simulink model "DBL_Master"  (R2020b)
settings: configuration reference "VLS_Standard_Configuration" (kept outside this file)
undefined symbols (not defined in the file): C_CSpeed0, C_DblDeadZone, C_DblInterDblAngValues, C_DblInterStwAngValues, C_DblRateLimit, C_DblSpeed0, C_LeftDblMaxAngle, C_LeftDblMinAngle, C_RightDblMaxAngle, C_RightDblMinAngle
libraries: DBL_MasterLib x1
settings Model: DataDictionary=DBL_Master_DD.sldd  EnableAccessToBaseWorkspace=off  Creator=mteama  LastModifiedBy=ahashem
settings ConfigSetRef: SourceName=VLS_Standard_Configuration

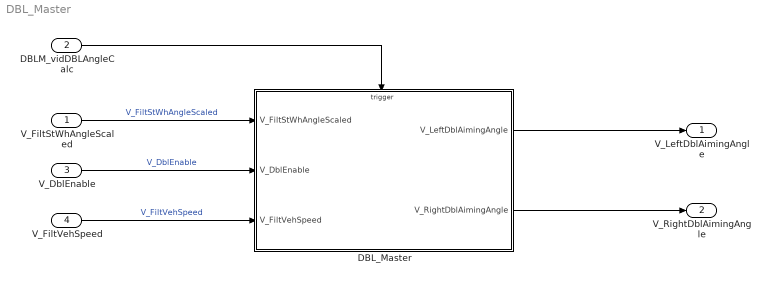
== system DBL_Master ==
  V_FiltStWhAngleScaled : Inport
  DBLM_vidDBLAngleCalc : Inport  Port=2  SampleTime=0.02  OutputFunctionCall=on
  V_DblEnable : Inport  Port=3
  V_FiltVehSpeed : Inport  Port=4
  DBL_Master : Subsystem  Description=DBLMasterLaw2 subsystem  TreatAsAtomicUnit=on
  V_LeftDblAimingAngle : Outport  VectorParamsAs1DForOutWhenUnconnected=off
  V_RightDblAimingAngle : Outport  Port=2  VectorParamsAs1DForOutWhenUnconnected=off
  wires:
  V_FiltStWhAngleScaled/1 -> DBL_Master/1(V_FiltStWhAngleScaled)  "V_FiltStWhAngleScaled"
  DBL_Master/1(V_LeftDblAimingAngle) -> V_LeftDblAimingAngle/1
  DBLM_vidDBLAngleCalc/1 -> DBL_Master/Trigger
  V_DblEnable/1 -> DBL_Master/2(V_DblEnable)  "V_DblEnable"
  V_FiltVehSpeed/1 -> DBL_Master/3(V_FiltVehSpeed)  "V_FiltVehSpeed"
  DBL_Master/2(V_RightDblAimingAngle) -> V_RightDblAimingAngle/1

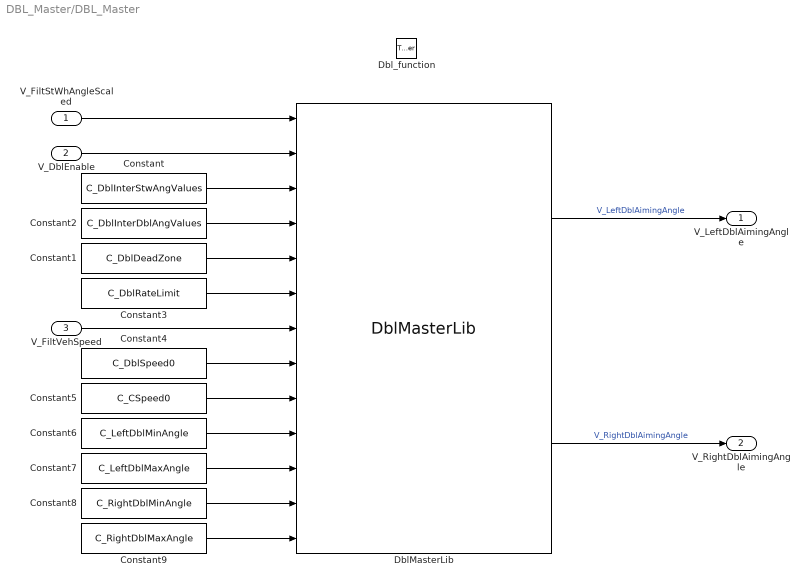
== system DBL_Master/DBL_Master ==
  V_FiltStWhAngleScaled : Inport
  V_DblEnable : Inport  Port=2
  V_FiltVehSpeed : Inport  Port=3
  Dbl_function : TriggerPort  TriggerType=function-call  VariantControl=Variant
      settings: AttributesFormatString=StatesWhenEnabling: %<StatesWhenEnabling>
  Constant : Constant  Value=C_DblInterStwAngValues  VectorParams1D=off
  Constant1 : Constant  Value=C_DblDeadZone  VectorParams1D=off
  Constant2 : Constant  Value=C_DblInterDblAngValues  VectorParams1D=off
  Constant3 : Constant  Value=C_DblRateLimit  VectorParams1D=off
  Constant4 : Constant  Value=C_DblSpeed0  VectorParams1D=off
  Constant5 : Constant  Value=C_CSpeed0  VectorParams1D=off
  Constant6 : Constant  Value=C_LeftDblMinAngle  VectorParams1D=off
  Constant7 : Constant  Value=C_LeftDblMaxAngle  VectorParams1D=off
  Constant8 : Constant  Value=C_RightDblMinAngle  VectorParams1D=off
  Constant9 : Constant  Value=C_RightDblMaxAngle  VectorParams1D=off
  DblMasterLib : DBL_MasterLib/DblMasterLib  SystemSampleTime=-1  VariantActivationTime=update diagram  Latency=0  AutoFrameSizeCalculation=off
  V_LeftDblAimingAngle : Outport  VectorParamsAs1DForOutWhenUnconnected=off
      settings: AttributesFormatString=OutputWhenDisabled: %<OutputWhenDisabled>
  V_RightDblAimingAngle : Outport  Port=2  VectorParamsAs1DForOutWhenUnconnected=off
      settings: AttributesFormatString=OutputWhenDisabled: %<OutputWhenDisabled>
  wires:
  DblMasterLib/1 -> V_LeftDblAimingAngle/1  "V_LeftDblAimingAngle"
  V_FiltStWhAngleScaled/1 -> DblMasterLib/1
  Constant/1 -> DblMasterLib/3
  Constant1/1 -> DblMasterLib/5
  Constant2/1 -> DblMasterLib/4
  V_DblEnable/1 -> DblMasterLib/2
  Constant3/1 -> DblMasterLib/6
  V_FiltVehSpeed/1 -> DblMasterLib/7
  Constant4/1 -> DblMasterLib/8
  Constant5/1 -> DblMasterLib/9
  Constant9/1 -> DblMasterLib/13
  Constant8/1 -> DblMasterLib/12
  Constant7/1 -> DblMasterLib/11
  Constant6/1 -> DblMasterLib/10
  DblMasterLib/2 -> V_RightDblAimingAngle/1  "V_RightDblAimingAngle"
